simulink model "fifio_with_fft"  (R2024a)
settings: Solver=FixedStepDiscrete  StartTime=0.0  StopTime=2  RelTol=1e-3
values from neighbouring files (symbols this model uses):
  enable_FIFO_in = Ts*1    (= 7.50007500075e-06)    [new_generation_coeff.m]
  enable_FIFO_out = Ts*9009    (= 0.0675681756818)    [new_generation_coeff.m]
  Finput = F_resolution*128    (= 260.4140625)    [new_generation_coeff.m]    (also in simon_test.m; testPSD_simulink.m)
  Ts = 1/Fs    (= 7.50007500075e-06)    [new_generation_coeff.m]    (also in simon_test.m; simple_fft_test.m = 1/F; testPSD_c2d.m; testPSD_simulink.m)
libraries: dsphdlxfrm2 x1, hdlsllib x1
settings Model: DataTypeOverride=Off  Creator=Simon  LastModifiedBy=Simon
settings OptimizationCC: BlockReduction=off  ConditionallyExecuteInputs=off  DefaultParameterBehavior=Inlined  InheritOutputTypeSmallerThanSingle=on
settings DebuggingCC: AlgebraicLoopMsg=error  SingleTaskRateTransMsg=error  UnconnectedInputMsg=warning  UnconnectedOutputMsg=warning  UnconnectedLineMsg=warning
settings HardwareCC: ProdBitPerPointer=32  ProdBitPerSizeT=32  ProdBitPerPtrDiffT=32  ProdLargestAtomicFloat=None  ProdIntDivRoundTo=Undefined  ProdEndianess=Unspecified  ProdWordSize=32  ProdHWDeviceType=ASIC/FPGA->ASIC/FPGA  TargetBitPerPointer=64  TargetBitPerSizeT=64  TargetBitPerPtrDiffT=64  TargetLongLongMode=on  TargetIntDivRoundTo=Zero  TargetEndianess=LittleEndian  TargetWordSize=64  TargetHWDeviceType=Custom Processor->MATLAB Host Computer  ProdEqTarget=off

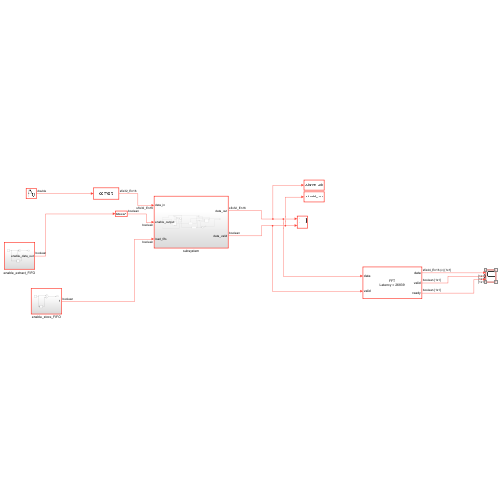
[thumbnail: Simulink's stored preview of the top-level diagram]
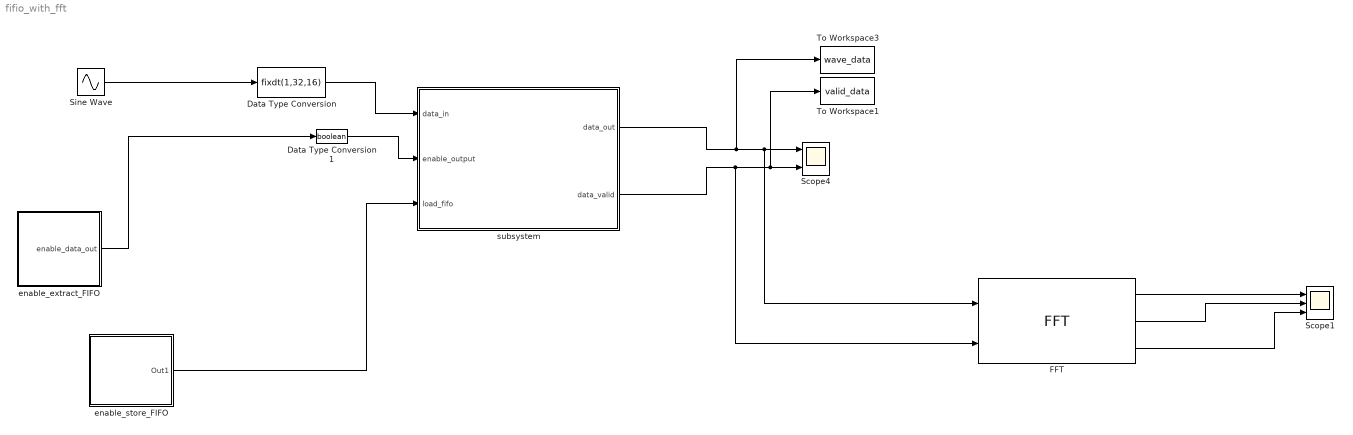
== system fifio_with_fft ==
  Data Type Conversion : DataTypeConversion  OutDataTypeStr=fixdt(1,32,16)  SaturateOnIntegerOverflow=off  RndMeth=Floor
  Data Type Conversion1 : DataTypeConversion  OutDataTypeStr=boolean  SaturateOnIntegerOverflow=off  RndMeth=Floor
  FFT : dsphdlxfrm2/FFT  Architecture=Burst Radix 2  FFTLengthSource=Property  FFTLength=4096  FFTLengthMax=1024  ComplexMultiplication=Use 4 multipliers and 2 adders  BitReversedOutput=off  BitReversedInput=off  Normalize=off  SimulateUsing=Code generation  RoundingMethod=Floor  ResetInputPort=off  StartOutputPort=off  EndOutputPort=off
  Scope1 : Scope  NumInputPorts=3
  Scope4 : Scope  NumInputPorts=2
  Sine Wave : Sin  Frequency=Finput*2*pi  Phase=2  SampleTime=Ts
  To Workspace1 : ToWorkspace  VariableName=valid_data  SampleTime=Ts
  To Workspace3 : ToWorkspace  VariableName=wave_data  SampleTime=Ts
  enable_extract_FIFO : Subsystem
  enable_store_FIFO : Subsystem
  subsystem : Subsystem
  wires:
  Sine Wave/1 -> Data Type Conversion/1
  enable_store_FIFO/1(Out1) -> subsystem/3(load_fifo)
  subsystem/1(data_out) -> To Workspace3/1, FFT/1, Scope4/1
  subsystem/2(data_valid) -> FFT/2, To Workspace1/1, Scope4/2
  Data Type Conversion/1 -> subsystem/1(data_in)
  enable_extract_FIFO/1(enable_data_out) -> Data Type Conversion1/1
  Data Type Conversion1/1 -> subsystem/2(enable_output)
  FFT/2 -> Scope1/2
  FFT/1 -> Scope1/1
  FFT/3 -> Scope1/3

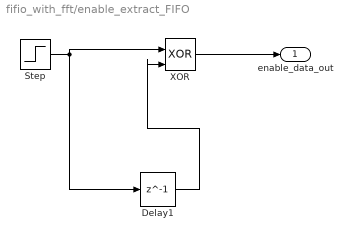
== system fifio_with_fft/enable_extract_FIFO ==
  Delay1 : Delay  DelayLength=1  InitialCondition=0  SampleTime=Ts
  Step : Step  Time=enable_FIFO_out  SampleTime=Ts
  XOR : Logic  Operator=XOR  IconShape=distinctive  AllPortsSameDT=off  OutDataTypeStr=boolean
  enable_data_out : Outport  OutDataTypeStr=boolean
  wires:
  Delay1/1 -> XOR/2
  Step/1 -> Delay1/1, XOR/1
  XOR/1 -> enable_data_out/1

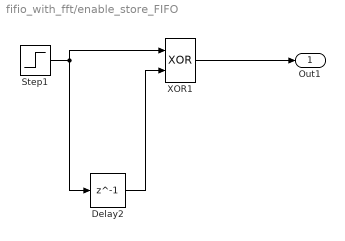
== system fifio_with_fft/enable_store_FIFO ==
  Delay2 : Delay  DelayLength=1  InitialCondition=0  SampleTime=Ts
  Step1 : Step  Time=enable_FIFO_in  SampleTime=Ts
  XOR1 : Logic  Operator=XOR  IconShape=distinctive  AllPortsSameDT=off  OutDataTypeStr=boolean
  Out1 : Outport  OutDataTypeStr=boolean
  wires:
  XOR1/1 -> Out1/1
  Step1/1 -> Delay2/1, XOR1/1
  Delay2/1 -> XOR1/2

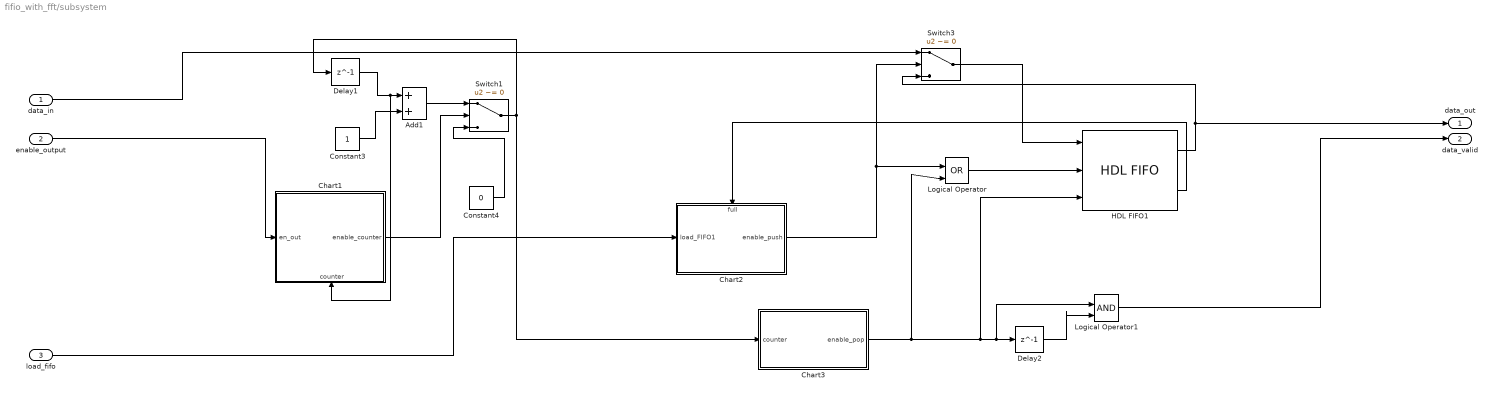
== system fifio_with_fft/subsystem ==
  data_in : Inport  OutDataTypeStr=fixdt(1,32,16)
  enable_output : Inport  Port=2  OutDataTypeStr=boolean
  load_fifo : Inport  Port=3  OutDataTypeStr=boolean
  Add1 : Sum  OutDataTypeStr=fixdt(0,13,0)
  Chart1 : Stateflow chart  TreatAsAtomicUnit=on
      settings: PortSchema="{\"entries\":[{\"content\":{\"sides\":[{\"content\":{\"connectorIds\":[\"In2\"]},\"type\":\"ConnectorPlacement.EquallySpacedRectSide\",\"uuid\":\"9d6f18ef-7bce-40b0-94a2-758e33355834\"},{\"content\":{\"connectorIds\":[\"Out1\"],\"side\":\"RIGHT\"},\"type\":\"ConnectorPlacement.EquallySpacedRectSide\",\"uuid\":\"7bab70ba-8111-4145-9c29-33f98ce79820\"},{\"content\":{\"side\":\"TOP\"},\"type\":\"ConnectorPlacement.EquallySpacedRectSide\",\"uuid\":\"d3288235-814f-4c71-bec2-04d07c53d63c\"},{\"content\":{\"connectorIds\":[\"In1\"],\"side\":\"BOTTOM\"},\"type\":\"ConnectorPlacement.EquallySpacedRectSide\",\"uuid\":\"018953e5-55f4-4114-8f5d-132f3f7565f7\"}]},\"type\":\"ConnectorPlacement.EquallySpacedConnector\",\"uuid\":\"70011da9-c6ae-4e69-953f-1d8cbe8c7c12\"}],\"packageUris\":[\"http://schema.mathworks.com/mf0/Connector/R2020b\"],\"version\":\"1.0\"}"
  Chart2 : Stateflow chart  TreatAsAtomicUnit=on
      settings: PortSchema="{\"entries\":[{\"content\":{\"sides\":[{\"content\":{\"connectorIds\":[\"In1\"]},\"type\":\"ConnectorPlacement.EquallySpacedRectSide\",\"uuid\":\"9d6f18ef-7bce-40b0-94a2-758e33355834\"},{\"content\":{\"connectorIds\":[\"Out1\"],\"side\":\"RIGHT\"},\"type\":\"ConnectorPlacement.EquallySpacedRectSide\",\"uuid\":\"7bab70ba-8111-4145-9c29-33f98ce79820\"},{\"content\":{\"connectorIds\":[\"In2\"],\"side\":\"TOP\"},\"type\":\"ConnectorPlacement.EquallySpacedRectSide\",\"uuid\":\"d3288235-814f-4c71-bec2-04d07c53d63c\"}]},\"type\":\"ConnectorPlacement.EquallySpacedConnector\",\"uuid\":\"70011da9-c6ae-4e69-953f-1d8cbe8c7c12\"}],\"packageUris\":[\"http://schema.mathworks.com/mf0/Connector/R2020b\"],\"version\":\"1.0\"}"
  Chart3 : Stateflow chart  TreatAsAtomicUnit=on
  Constant3 : Constant  OutDataTypeStr=fixdt(0,12,0)  SampleTime=Ts
  Constant4 : Constant  Value=0  OutDataTypeStr=fixdt(1,13,0)  SampleTime=Ts
  Delay1 : Delay  DelayLength=1  InitialCondition=0  SampleTime=Ts
  Delay2 : Delay  DelayLength=1  InitialCondition=0  SampleTime=Ts
  HDL FIFO1 : hdlsllib/HDL RAMs/HDL FIFO  fifo_size=4096  mode=Classic  ratio=1  push_msg=Warning  pop_msg=Warning  show_empty=off  show_full=on  show_num=off  LabelModeActiveChoice_Mode=Classic  rst_port=off
  Logical Operator : Logic  Operator=OR  IconShape=distinctive  AllPortsSameDT=off  OutDataTypeStr=boolean
  Logical Operator1 : Logic  IconShape=distinctive  AllPortsSameDT=off  OutDataTypeStr=boolean
  Switch1 : Switch  Criteria=u2 ~= 0  OutDataTypeStr=fixdt(0,13,0)  SaturateOnIntegerOverflow=off  InputSameDT=off
  Switch3 : Switch  Criteria=u2 ~= 0  OutDataTypeStr=fixdt(1,32,16)  SaturateOnIntegerOverflow=off  InputSameDT=off
  data_out : Outport  OutDataTypeStr=fixdt(1,32,16)
  data_valid : Outport  Port=2
  wires:
  Delay1/1 -> Chart1/1(counter), Add1/1
  Logical Operator/1 -> HDL FIFO1/2
  HDL FIFO1/1 -> data_out/1, Switch3/3
  Switch1/1 -> Chart3/1(counter), Delay1/1
  Delay2/1 -> Logical Operator1/2
  enable_output/1 -> Chart1/2(en_out)
  Add1/1 -> Switch1/1
  Constant3/1 -> Add1/2
  HDL FIFO1/2 -> Chart2/2(full)
  Switch3/1 -> HDL FIFO1/1
  Constant4/1 -> Switch1/3
  Logical Operator1/1 -> data_valid/1
  load_fifo/1 -> Chart2/1(load_FIFO1)
  data_in/1 -> Switch3/1
  Chart3/1(enable_pop) -> HDL FIFO1/3, Logical Operator1/1, Delay2/1, Logical Operator/2
  Chart1/1(enable_counter) -> Switch1/2
  Chart2/1(enable_push) -> Switch3/2, Logical Operator/1

== stateflow chart fifio_with_fft/subsystem/Chart1 ==
  settings: updateMethod=DISCRETE  sampleTime=Ts  executeAtInitialization=1
  state initial_counter
    during:
    enable_counter = false;
  state counter_state
    during:
    enable_counter = true;
  (default) -> initial_counter
  counter_state -> initial_counter : [counter == 1+4096]
  initial_counter -> counter_state : [en_out == true]
  data: counter input fixdt(0,13,0); enable_counter output boolean; en_out input boolean

== stateflow chart fifio_with_fft/subsystem/Chart2 ==
  settings: updateMethod=DISCRETE  sampleTime=Ts  executeAtInitialization=1
  state initial_push
    during:
    enable_push = false;
  state push_state
    during:
    enable_push = true;
  (default) -> initial_push
  push_state -> initial_push : [full == true]
  initial_push -> push_state : [load_FIFO1 == true]
  data: load_FIFO1 input boolean; full input boolean; enable_push output boolean

== stateflow chart fifio_with_fft/subsystem/Chart3 ==
  settings: updateMethod=DISCRETE  sampleTime=Ts  executeAtInitialization=1
  state initial_popstate
    during:
    enable_pop = false;
  state pop_state
    during:
    enable_pop = true;
  (default) -> initial_popstate
  pop_state -> initial_popstate : [counter == 2+4096]
  initial_popstate -> pop_state : [counter == 1]
  data: enable_pop output boolean; counter input fixdt(0,13,0)
